simulink model "sampleModel1619"  (R2023a)
settings: Solver=VariableStepAuto  StartTime=0.0  StopTime=10.0  RelTol=1e-3
libraries: hdlsllib x4, simulink x2
settings Model: Creator=user1  LastModifiedBy=user1

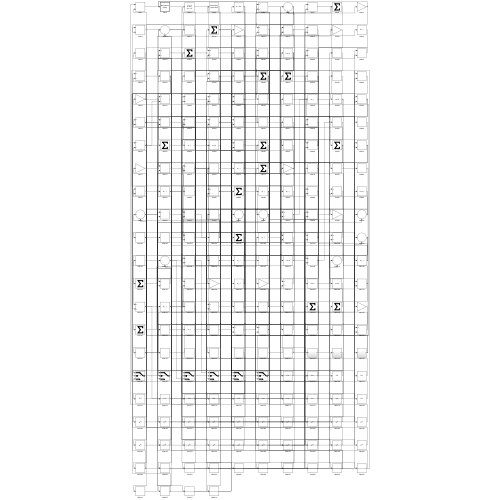
[thumbnail: Simulink's stored preview of the top-level diagram]
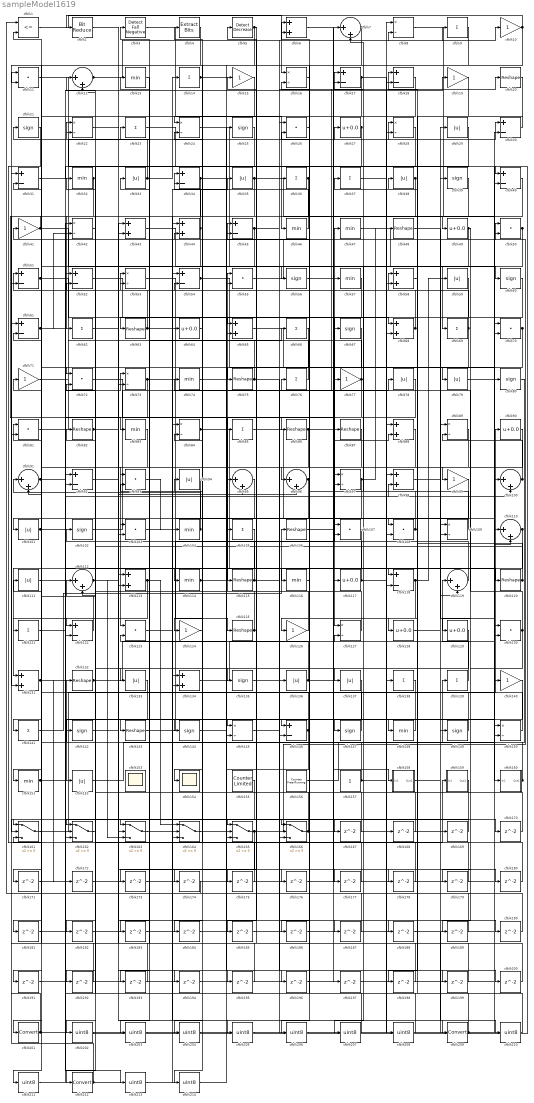
== system sampleModel1619 ==
  cfblk1 : RelationalOperator  Operator=<=  OutDataTypeStr=boolean  InputSameDT=off
  cfblk{10,15,19,41,71,77,99,124,126,140} (10 alike) : Gain
  cfblk{7,12,91,95..96,100,110,112,119} (9 alike) : Sum  Inputs=|++
  cfblk{29,33,35,38,59,78..79,94,101,111,133,136..137,152} (14 alike) : Abs  SaturateOnIntegerOverflow=off
  cfblk{21,25,39,56,60,67,80,102,135,142,144,147,149} (13 alike) : Signum
  cfblk{11,26,50,55,70,72,81,93,103,107..108,123,130} (13 alike) : DotProduct  OutDataTypeStr=Inherit: Inherit via internal rule
  cfblk{13,32,46..47,57,74,83,104,114,116,148,151} (12 alike) : MinMax
  cfblk{9,14,23,36..37,62,66,69,76,85,105,121,138..139,141} (15 alike) : Sum  Inputs=+
  cfblk{20,48,63,75,82,86..87,106,115,120,125,132,143} (13 alike) : Reshape
  cfblk{8,16,22,24,28,42,53,73,84,89,97,109,127,145,150} (15 alike) : Product  Inputs=*/  RndMeth=Zero  SaturateOnIntegerOverflow=on
  cfblk{6,43..44,58,65,68,88,98,113,131,134} (11 alike) : Sum
  cfblk{27,49,64,90,117,128..129} (7 alike) : Bias  Bias=0.0  SaturateOnIntegerOverflow=off
  cfblk{17..18,30..31,34,40,45,51..52,54,61,92,118,122,146} (15 alike) : Sum  Inputs=+-
  cfblk153 : Scope
      settings: Floating=on
  cfblk154 : Scope
  cfblk155 : hdlsllib/Sources/Counter Limited  uplimit=7  tsamp=-1
  cfblk156 : hdlsllib/Sources/Counter Free-Running  NumBits=16  tsamp=-1
  cfblk157 : Constant  SampleTime=-1
  cfblk158 : Subsystem
      settings: LibrarySourceBlock=|
      | hdlsllib/Ports &
      | Subsystems/Subsystem
  cfblk159 : Subsystem
      settings: LibrarySourceBlock=|
      | hdlsllib/Ports &
      | Subsystems/Subsystem
  cfblk160 : Subsystem
      settings: LibrarySourceBlock=|
      | hdlsllib/Ports &
      | Subsystems/Subsystem
  cfblk{161..166} (6 alike) : Switch  SaturateOnIntegerOverflow=off  InputSameDT=off
  cfblk{167..200} (34 alike) : Delay  SampleTime=1
  cfblk2 : hdlsllib/Logic and Bit Operations/Bit Reduce  mode=AND
  cfblk201 : DataTypeConversion  SaturateOnIntegerOverflow=off  RndMeth=Floor
  cfblk{202..208,210..211,213..214} (11 alike) : DataTypeConversion  OutDataTypeStr=uint8  SaturateOnIntegerOverflow=off  RndMeth=Floor
  cfblk209 : DataTypeConversion  SaturateOnIntegerOverflow=off  RndMeth=Floor
  cfblk212 : DataTypeConversion  SaturateOnIntegerOverflow=off  RndMeth=Floor
  cfblk3 : hdlsllib/Logic and Bit Operations/Detect Fall Negative  vinit=0  OutDataTypeStr=boolean
  cfblk4 : simulink/Logic and Bit Operations/Extract Bits  bitsToExtract=Upper half  numBits=8  bitIdxRange=[0 7]  outScalingMode=Preserve fixed-point scaling
      settings: LibrarySourceBlock=|
      | hdlsllib/Logic and Bit
      | Operations/Extract Bits
  cfblk5 : simulink/Logic and Bit Operations/Detect Decrease  vinit=0.0  OutDataTypeStr=boolean
      settings: LibrarySourceBlock=|
      | hdlsllib/Logic and Bit
      | Operations/Detect
      | Decrease
  wires:
  cfblk57/1 -> cfblk127/1
  cfblk75/1 -> cfblk34/2, cfblk200/1
  cfblk92/1 -> cfblk209/1
  cfblk80/1 -> cfblk132/1
  cfblk102/1 -> cfblk20/1
  cfblk14/1 -> cfblk166/3, cfblk199/1
  cfblk108/1 -> cfblk41/1, cfblk57/1, cfblk198/1
  cfblk15/1 -> cfblk24/1
  cfblk141/1 -> cfblk106/1
  cfblk95/1 -> cfblk212/1
  cfblk165/1 -> cfblk50/1, cfblk193/1
  cfblk71/1 -> cfblk28/1
  cfblk161/1 -> cfblk90/1
  cfblk35/1 -> cfblk49/1, cfblk133/1, cfblk17/2, cfblk164/2
  cfblk109/1 -> cfblk76/1
  cfblk85/1 -> cfblk117/1
  cfblk3/1 -> cfblk46/1
  cfblk73/1 -> cfblk125/1, cfblk122/2, cfblk85/1, cfblk187/1
  cfblk134/1 -> cfblk70/1
  cfblk127/1 -> cfblk55/1
  cfblk105/1 -> cfblk131/1
  cfblk28/1 -> cfblk154/1
  cfblk41/1 -> cfblk83/1, cfblk64/1
  cfblk93/1 -> cfblk104/1
  cfblk21/1 -> cfblk159/1(In1)
  cfblk30/1 -> cfblk37/1
  cfblk143/1 -> cfblk47/1
  cfblk89/1 -> cfblk99/1
  cfblk24/1 -> cfblk69/1
  cfblk79/1 -> cfblk130/1
  cfblk53/1 -> cfblk140/1
  cfblk64/1 -> cfblk114/1
  cfblk160/1(Out1) -> cfblk111/1, cfblk53/2
  cfblk55/1 -> cfblk7/1
  cfblk66/1 -> cfblk165/1
  cfblk162/1 -> cfblk102/1
  cfblk113/1 -> cfblk121/1, cfblk164/1
  cfblk150/1 -> cfblk32/1
  cfblk83/1 -> cfblk123/1
  cfblk148/1 -> cfblk143/1
  cfblk44/1 -> cfblk34/1, cfblk141/1
  cfblk36/1 -> cfblk135/1, cfblk81/2
  cfblk72/1 -> cfblk115/1
  cfblk68/1 -> cfblk63/1, cfblk12/2, cfblk22/1
  cfblk107/1 -> cfblk146/1
  cfblk19/1 -> cfblk118/1
  cfblk1/1 -> cfblk16/1
  cfblk77/1 -> cfblk23/1, cfblk17/1, cfblk103/2
  cfblk11/1 -> cfblk70/2
  cfblk16/1 -> cfblk36/1
  cfblk12/1 -> cfblk10/1, cfblk177/1
  cfblk126/1 -> cfblk33/1
  cfblk87/1 -> cfblk144/1
  cfblk32/1 -> cfblk62/1, cfblk51/2
  cfblk33/1 -> cfblk14/1, cfblk21/1
  cfblk84/1 -> cfblk120/1, cfblk50/2
  cfblk69/1 -> cfblk137/1, cfblk7/2, cfblk162/2
  cfblk17/1 -> cfblk190/1, cfblk191/1
  cfblk39/1 -> cfblk96/1
  cfblk119/1 -> cfblk15/1
  cfblk131/1 -> cfblk100/2, cfblk172/1
  cfblk116/1 -> cfblk6/1
  cfblk6/1 -> cfblk158/1(In1)
  cfblk149/1 -> cfblk71/1
  cfblk97/1 -> cfblk107/1, cfblk48/1
  cfblk22/1 -> cfblk96/2
  cfblk147/1 -> cfblk105/1
  cfblk67/1 -> cfblk145/1
  cfblk145/1 -> cfblk127/2
  cfblk7/1 -> cfblk124/1, cfblk175/1
  cfblk18/1 -> cfblk97/2
  cfblk78/1 -> cfblk116/1
  cfblk156/1 -> cfblk139/1
  cfblk54/1 -> cfblk79/1, cfblk56/1
  cfblk110/1 -> cfblk113/2, cfblk203/1
  cfblk111/1 -> cfblk147/1
  cfblk42/1 -> cfblk12/1
  cfblk63/1 -> cfblk87/1, cfblk31/2
  cfblk157/1 -> cfblk28/2, cfblk61/2
  cfblk27/1 -> cfblk52/1, cfblk103/1, cfblk162/3
  cfblk59/1 -> cfblk148/1
  cfblk45/1 -> cfblk27/1, cfblk91/2
  cfblk8/1 -> cfblk110/1
  cfblk135/1 -> cfblk9/1
  cfblk91/1 -> cfblk42/1, cfblk213/1
  cfblk52/1 -> cfblk65/1
  cfblk114/1 -> cfblk94/1, cfblk77/1
  cfblk159/1(Out1) -> cfblk166/1
  cfblk38/1 -> cfblk131/2, cfblk73/2
  cfblk10/1 -> cfblk145/2, cfblk2/1
  cfblk23/1 -> cfblk107/2
  cfblk51/1 -> cfblk134/1, cfblk119/2
  cfblk140/1 -> cfblk152/1
  cfblk130/1 -> cfblk74/1, cfblk179/1
  cfblk104/1 -> cfblk13/1, cfblk91/1
  cfblk86/1 -> cfblk88/2, cfblk165/3, cfblk164/3
  cfblk120/1 -> cfblk18/1, cfblk22/2
  cfblk48/1 -> cfblk130/2
  cfblk88/1 -> cfblk161/1
  cfblk81/1 -> cfblk55/2
  cfblk136/1 -> cfblk8/2, cfblk45/2, cfblk3/1
  cfblk99/1 -> cfblk101/1
  cfblk132/1 -> cfblk25/1, cfblk66/1
  cfblk164/1 -> cfblk30/1
  cfblk100/1 -> cfblk93/1, cfblk89/2
  cfblk43/1 -> cfblk80/1
  cfblk9/1 -> cfblk86/1
  cfblk125/1 -> cfblk93/2, cfblk51/1
  cfblk62/1 -> cfblk68/1
  cfblk166/1 -> cfblk149/1, cfblk4/1
  cfblk98/1 -> cfblk29/1
  cfblk20/1 -> cfblk128/1
  cfblk40/1 -> cfblk201/1
  cfblk50/1 -> cfblk122/1, cfblk192/1
  cfblk31/1 -> cfblk19/1
  cfblk76/1 -> cfblk44/2
  cfblk58/1 -> cfblk108/1
  cfblk94/1 -> cfblk134/2
  cfblk46/1 -> cfblk24/2
  cfblk115/1 -> cfblk166/2, cfblk84/2, cfblk82/1
  cfblk146/1 -> cfblk45/1, cfblk165/2
  cfblk128/1 -> cfblk39/1
  cfblk70/1 -> cfblk129/1, cfblk181/1
  cfblk152/1 -> cfblk30/2
  cfblk65/1 -> cfblk160/1(In1)
  cfblk133/1 -> cfblk162/1
  cfblk25/1 -> cfblk163/1
  cfblk123/1 -> cfblk78/1
  cfblk118/1 -> cfblk58/1, cfblk126/1, cfblk59/1
  cfblk82/1 -> cfblk194/1, cfblk195/1
  cfblk34/1 -> cfblk72/1, cfblk196/1, cfblk214/1
  cfblk122/1 -> cfblk81/1
  cfblk96/1 -> cfblk184/1, cfblk185/1
  cfblk151/1 -> cfblk142/1, cfblk98/2
  cfblk5/1 -> cfblk75/1, cfblk11/2
  cfblk112/1 -> cfblk43/2, cfblk163/3
  cfblk103/1 -> cfblk35/1
  cfblk61/1 -> cfblk150/2, cfblk42/2
  cfblk139/1 -> cfblk119/1
  cfblk101/1 -> cfblk73/1, cfblk151/1
  cfblk158/1(Out1) -> cfblk109/2
  cfblk49/1 -> cfblk67/1, cfblk189/1
  cfblk117/1 -> cfblk98/1, cfblk53/1
  cfblk47/1 -> cfblk60/1
  cfblk121/1 -> cfblk167/1
  cfblk167/1 -> cfblk112/2
  cfblk168/1 -> cfblk113/1
  cfblk169/1 -> cfblk161/2
  cfblk144/1 -> cfblk170/1
  cfblk170/1 -> cfblk88/1
  cfblk4/1 -> cfblk171/1
  cfblk171/1 -> cfblk68/2
  cfblk172/1 -> cfblk44/1
  cfblk13/1 -> cfblk173/1
  cfblk173/1 -> cfblk100/1
  cfblk124/1 -> cfblk174/1
  cfblk174/1 -> cfblk1/1
  cfblk175/1 -> cfblk84/1
  cfblk2/1 -> cfblk176/1
  cfblk176/1 -> cfblk97/1
  cfblk177/1 -> cfblk52/2
  cfblk74/1 -> cfblk178/1
  cfblk178/1 -> cfblk16/2
  cfblk179/1 -> cfblk163/2
  cfblk56/1 -> cfblk180/1
  cfblk180/1 -> cfblk54/2
  cfblk181/1 -> cfblk65/2
  cfblk129/1 -> cfblk182/1
  cfblk182/1 -> cfblk146/2
  cfblk137/1 -> cfblk183/1
  cfblk183/1 -> cfblk8/1
  cfblk184/1 -> cfblk89/1
  cfblk185/1 -> cfblk18/2
  cfblk29/1 -> cfblk186/1
  cfblk186/1 -> cfblk150/1
  cfblk187/1 -> cfblk72/2
  cfblk142/1 -> cfblk188/1
  cfblk189/1 -> cfblk6/2
  cfblk190/1 -> cfblk109/1
  cfblk191/1 -> cfblk118/2
  cfblk192/1 -> cfblk161/3
  cfblk193/1 -> cfblk1/2
  cfblk194/1 -> cfblk58/2
  cfblk195/1 -> cfblk123/2
  cfblk196/1 -> cfblk108/2
  cfblk106/1 -> cfblk197/1
  cfblk197/1 -> cfblk110/2
  cfblk198/1 -> cfblk31/1
  cfblk199/1 -> cfblk43/1
  cfblk200/1 -> cfblk5/1
  cfblk201/1 -> cfblk169/1, cfblk61/1
  cfblk155/1 -> cfblk202/1
  cfblk202/1 -> cfblk40/1
  cfblk203/1 -> cfblk40/2
  cfblk138/1 -> cfblk204/1
  cfblk204/1 -> cfblk136/1
  cfblk163/1 -> cfblk205/1
  cfblk205/1 -> cfblk138/1
  cfblk26/1 -> cfblk206/1
  cfblk206/1 -> cfblk168/1
  cfblk60/1 -> cfblk207/1
  cfblk207/1 -> cfblk26/1
  cfblk37/1 -> cfblk208/1
  cfblk208/1 -> cfblk26/2
  cfblk209/1 -> cfblk38/1, cfblk112/1
  cfblk188/1 -> cfblk210/1
  cfblk210/1 -> cfblk92/1
  cfblk90/1 -> cfblk211/1
  cfblk211/1 -> cfblk92/2
  cfblk212/1 -> cfblk11/1, cfblk54/1
  cfblk213/1 -> cfblk95/1
  cfblk214/1 -> cfblk95/2

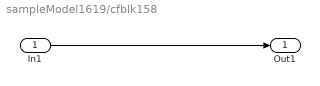
== system sampleModel1619/cfblk158 ==
  In1 : Inport
  Out1 : Outport
  wires:
  In1/1 -> Out1/1

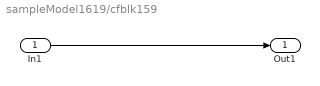
== system sampleModel1619/cfblk159 ==
  In1 : Inport
  Out1 : Outport
  wires:
  In1/1 -> Out1/1

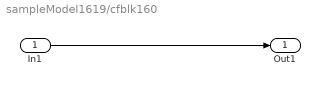
== system sampleModel1619/cfblk160 ==
  In1 : Inport
  Out1 : Outport
  wires:
  In1/1 -> Out1/1
